simulink subsystem "vector_from_bus"  (R2024a)
settings: Solver=VariableStepAuto  StartTime=0.0  StopTime=10.0  RelTol=1e-3
settings Model: Creator=Friedrich Tuttas  LastModifiedBy=Friedrich Tuttas

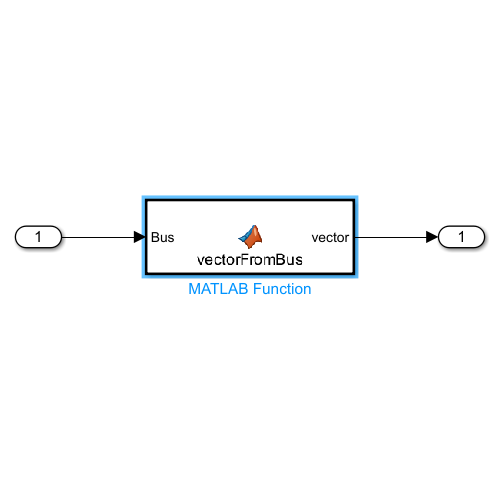
[thumbnail: Simulink's stored preview of the top-level diagram]
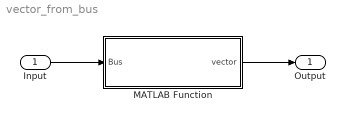
== system vector_from_bus ==
  Input : Inport
  MATLAB Function : MATLAB Function  TreatAsAtomicUnit=on
  Output : Outport
  wires:
  Input/1 -> MATLAB Function/1(Bus)
  MATLAB Function/1(vector) -> Output/1

== matlab function vector_from_bus/MATLAB Function ==
  data: Bus input; vector output
function vector = vectorFromBus(Bus)


[vector, ~] = populateVectorFromNumericStructure(Bus);

end
